simulink model "PID_systems"  (R2018a)
settings: Solver=VariableStepAuto  StartTime=0.0  StopTime=15  FixedStep=0.05  RelTol=1e-3
values from neighbouring files (symbols this model uses):
  Kd = -0.7    [pid_parameter_sweep.m]
  Ki = 0    [pid_parameter_sweep.m]
  Kp = -2.2    [pid_parameter_sweep.m]
libraries: slident x1
settings Model: Creator=Zeljko  LastModifiedBy=Zeljko
settings SolverCC: ZeroCrossAlgorithm=Adaptive
settings DebuggingCC: MaxConsecutiveZCsMsg=none

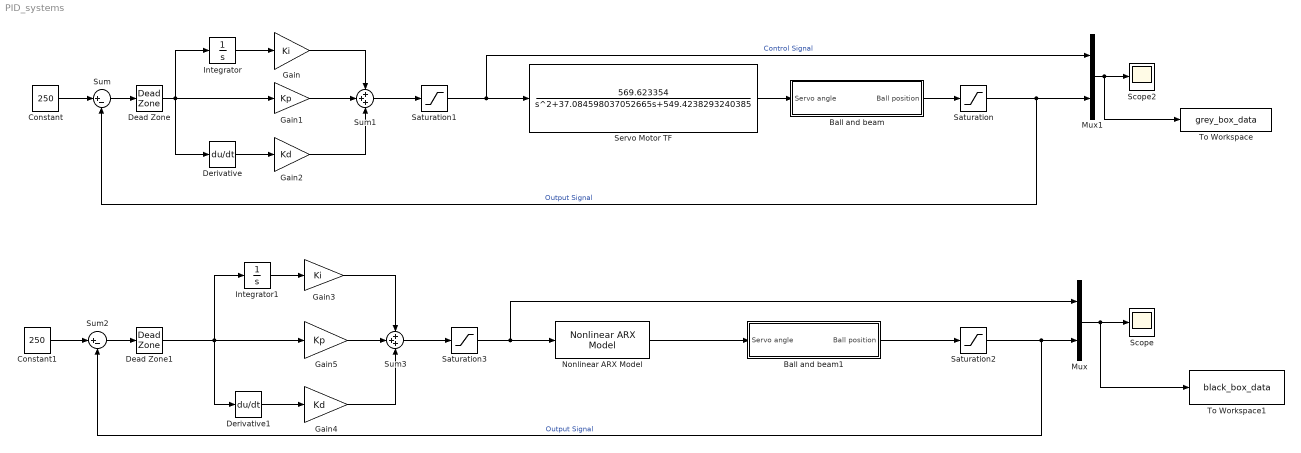
== system PID_systems ==
  Ball and beam : Subsystem
  Ball and beam1 : Subsystem
  Constant : Constant  Value=250
  Constant1 : Constant  Value=250
  Dead Zone : DeadZone  LowerValue=-5  UpperValue=5  ZeroCross=off  SaturateOnIntegerOverflow=on
  Dead Zone1 : DeadZone  LowerValue=-5  UpperValue=5  ZeroCross=off  SaturateOnIntegerOverflow=on
  Derivative : Derivative
  Derivative1 : Derivative
  Gain : Gain  Gain=Ki
  Gain1 : Gain  Gain=Kp
  Gain2 : Gain  Gain=Kd
  Gain3 : Gain  Gain=Ki
  Gain4 : Gain  Gain=Kd
  Gain5 : Gain  Gain=Kp
  Integrator : Integrator
  Integrator1 : Integrator
  Mux : Mux  Inputs=2
  Mux1 : Mux  Inputs=2
  Nonlinear ARX Model : slident/Models/Nonlinear ARX Model  sys=sys  ICspec=State values  X0=[0;0;0;0;0;0;0]  U0=0  Y0=0
      settings: SourceProductName=System Identification Toolbox  SourceProductBaseCode=ID
  Saturation : Saturate  UpperLimit=400  LowerLimit=0  ZeroCross=off
  Saturation1 : Saturate  UpperLimit=45  LowerLimit=-45  ZeroCross=off
  Saturation2 : Saturate  UpperLimit=400  LowerLimit=0  ZeroCross=off
  Saturation3 : Saturate  UpperLimit=45  LowerLimit=-45  ZeroCross=off
  Scope : Scope
  Scope2 : Scope
  Servo Motor TF : TransferFcn  Numerator=569.623354  Denominator=[1, 37.084598037052665, 549.4238293240385]
  Sum : Sum  Inputs=|+-
  Sum1 : Sum  Inputs=+++
  Sum2 : Sum  Inputs=|+-
  Sum3 : Sum  Inputs=+++
  To Workspace : ToWorkspace  VariableName=grey_box_data  SaveFormat=Timeseries  SampleTime=-1
  To Workspace1 : ToWorkspace  VariableName=black_box_data  SaveFormat=Timeseries  SampleTime=-1
  wires:
  Constant/1 -> Sum/1
  Ball and beam/1(Ball position) -> Saturation/1
  Saturation/1 -> Mux1/2, Sum/2  "Output Signal"
  Saturation1/1 -> Mux1/1, Servo Motor TF/1  "Control Signal"
  Derivative/1 -> Gain2/1
  Integrator/1 -> Gain/1
  Sum/1 -> Dead Zone/1
  Gain/1 -> Sum1/1
  Gain1/1 -> Sum1/2
  Gain2/1 -> Sum1/3
  Servo Motor TF/1 -> Ball and beam/1(Servo angle)
  Sum1/1 -> Saturation1/1
  Mux1/1 -> To Workspace/1, Scope2/1
  Dead Zone/1 -> Derivative/1, Gain1/1, Integrator/1
  Gain5/1 -> Sum3/2
  Saturation3/1 -> Mux/1, Nonlinear ARX Model/1
  Nonlinear ARX Model/1 -> Ball and beam1/1(Servo angle)
  Gain3/1 -> Sum3/1
  Sum3/1 -> Saturation3/1
  Integrator1/1 -> Gain3/1
  Derivative1/1 -> Gain4/1
  Gain4/1 -> Sum3/3
  Ball and beam1/1(Ball position) -> Saturation2/1
  Sum2/1 -> Dead Zone1/1
  Saturation2/1 -> Mux/2, Sum2/2  "Output Signal"
  Mux/1 -> To Workspace1/1, Scope/1
  Constant1/1 -> Sum2/1
  Dead Zone1/1 -> Integrator1/1, Gain5/1, Derivative1/1

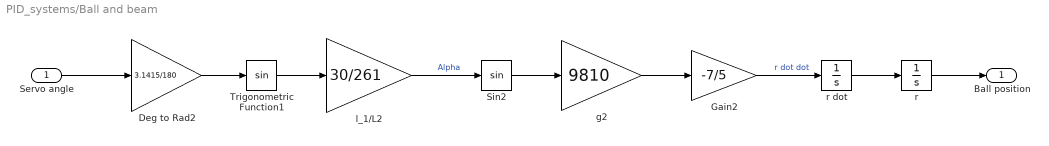
== system PID_systems/Ball and beam ==
  Servo angle : Inport
  Deg to Rad2 : Gain  Gain=3.1415/180
  Gain2 : Gain  Gain=-7/5
  Sin2 : Trigonometry
  Trigonometric Function1 : Trigonometry
  g2 : Gain  Gain=9810
  l_1/L2 : Gain  Gain=30/261
  r : Integrator  InitialCondition=100
  r dot : Integrator
  Ball position : Outport
  wires:
  g2/1 -> Gain2/1
  Sin2/1 -> g2/1
  Deg to Rad2/1 -> Trigonometric Function1/1
  r dot/1 -> r/1
  l_1/L2/1 -> Sin2/1  "Alpha"
  Trigonometric Function1/1 -> l_1/L2/1
  Gain2/1 -> r dot/1  "r dot dot"
  r/1 -> Ball position/1
  Servo angle/1 -> Deg to Rad2/1

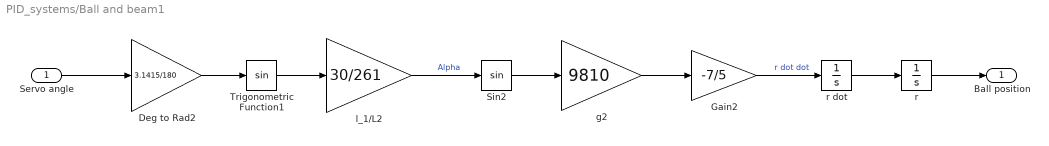
== system PID_systems/Ball and beam1 ==
  Servo angle : Inport
  Deg to Rad2 : Gain  Gain=3.1415/180
  Gain2 : Gain  Gain=-7/5
  Sin2 : Trigonometry
  Trigonometric Function1 : Trigonometry
  g2 : Gain  Gain=9810
  l_1/L2 : Gain  Gain=30/261
  r : Integrator  InitialCondition=100
  r dot : Integrator
  Ball position : Outport
  wires:
  g2/1 -> Gain2/1
  Sin2/1 -> g2/1
  Deg to Rad2/1 -> Trigonometric Function1/1
  r dot/1 -> r/1
  l_1/L2/1 -> Sin2/1  "Alpha"
  Trigonometric Function1/1 -> l_1/L2/1
  Gain2/1 -> r dot/1  "r dot dot"
  r/1 -> Ball position/1
  Servo angle/1 -> Deg to Rad2/1
